simulink library "StarTracker"  (R2014b)
settings: Solver=VariableStepAuto  StartTime=0.0  StopTime=10.0  RelTol=1e-3
undefined symbols (not defined in the file): ConfParam
libraries: simulink x2, Qprod x2, Normalization x1
settings Model: Creator=y.akisheva  LastModifiedBy=Hp
settings DataIOCC: SaveFormat=Dataset
settings OptimizationCC: UseDivisionForNetSlopeComputation=off  SimCompilerOptimization=off
settings DebuggingCC: SolverPrmCheckMsg=none  FrameProcessingCompatibilityMsg=error  AllowSymbolicDim=off
settings HardwareCC: ProdBitPerPointer=64  ProdLargestAtomicFloat=Float  ProdIntDivRoundTo=Zero  ProdEndianess=LittleEndian  ProdWordSize=64  ProdHWDeviceType=Intel->x86-64 (Windows64)
settings RTWCC: RTWCompilerOptimization=off
settings GRTTargetCC: GeneratePreprocessorConditionals=Use local settings
settings ConfigComp: CovMetricSettings=dw  CovHtmlReporting=on  CovSaveCumulativeToWorkspaceVar=on  CovSaveSingleToWorkspaceVar=on  CovExternalEMLEnable=off

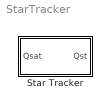
== system StarTracker ==
  Star Tracker : Subsystem

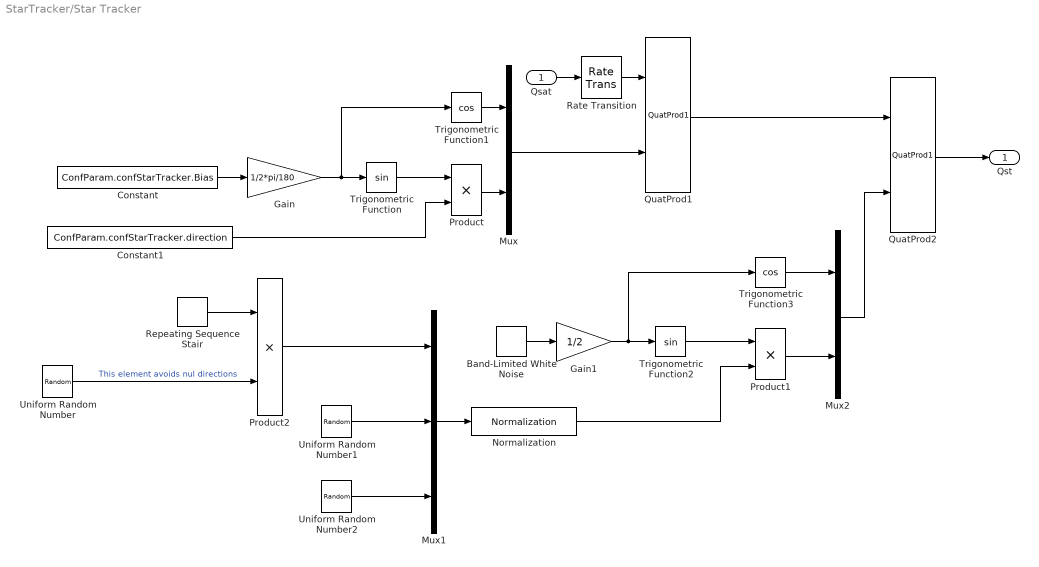
== system StarTracker/Star Tracker ==
  Qsat : Inport
  Band-Limited White Noise : simulink/Sources/Band-Limited White Noise  Cov=ConfParam.confStarTracker.NoisePower  Ts=1/ConfParam.confStarTracker.frequency  seed=[23341]
  Constant : Constant  Value=ConfParam.confStarTracker.Bias  SampleTime=1/ConfParam.confStarTracker.frequency
  Constant1 : Constant  Value=ConfParam.confStarTracker.direction  SampleTime=1/ConfParam.confStarTracker.frequency
  Gain : Gain  Gain=1/2*pi/180
  Gain1 : Gain  Gain=1/2
  Mux : Mux  Inputs=2
  Mux1 : Mux  Inputs=3
  Mux2 : Mux  Inputs=2
  Normalization : Normalization/Normalization
  Product : Product
  Product1 : Product
  Product2 : Product
  QuatProd1 : Qprod/QuatProd1
  QuatProd2 : Qprod/QuatProd1
  Rate Transition : RateTransition  X0=ConfParam.confStarTracker.InitQsat  OutPortSampleTime=1/ConfParam.confStarTracker.frequency
  Repeating Sequence Stair : simulink/Sources/Repeating Sequence Stair  OutValues=[1 -1].'  tsamp=1/ConfParam.confStarTracker.frequency  OutMin=[]  OutMax=[]  OutDataTypeStr=double  OutputDataTypeScalingMode=double  OutDataType=fixdt(0,8)  ConRadixGroup=Best Precision: Vector-wise  OutScaling=2^-12
  Trigonometric Function : Trigonometry
  Trigonometric Function1 : Trigonometry  Operator=cos
  Trigonometric Function2 : Trigonometry
  Trigonometric Function3 : Trigonometry  Operator=cos
  Uniform Random Number : UniformRandomNumber  Minimum=0.001  Maximum=1.001  SampleTime=1/ConfParam.confStarTracker.frequency
  Uniform Random Number1 : UniformRandomNumber  SampleTime=1/ConfParam.confStarTracker.frequency
  Uniform Random Number2 : UniformRandomNumber  SampleTime=1/ConfParam.confStarTracker.frequency
  Qst : Outport
  wires:
  QuatProd2/1 -> Qst/1
  Constant/1 -> Gain/1
  Trigonometric Function/1 -> Product/1
  Constant1/1 -> Product/2
  Gain/1 -> Trigonometric Function1/1, Trigonometric Function/1
  Product/1 -> Mux/2
  Trigonometric Function1/1 -> Mux/1
  Rate Transition/1 -> QuatProd1/1
  Band-Limited White Noise/1 -> Gain1/1
  Uniform Random Number1/1 -> Mux1/2
  Uniform Random Number/1 -> Product2/2  "This element avoids nul directions"
  Uniform Random Number2/1 -> Mux1/3
  Mux1/1 -> Normalization/1
  Trigonometric Function2/1 -> Product1/1
  Normalization/1 -> Product1/2
  QuatProd1/1 -> QuatProd2/1
  Product1/1 -> Mux2/2
  Trigonometric Function3/1 -> Mux2/1
  Mux2/1 -> QuatProd2/2
  Gain1/1 -> Trigonometric Function3/1, Trigonometric Function2/1
  Qsat/1 -> Rate Transition/1
  Mux/1 -> QuatProd1/2
  Repeating Sequence Stair/1 -> Product2/1
  Product2/1 -> Mux1/1
